simulink model "MTotalRequested"  (R2024b)
settings: Solver=FixedStepAuto  StartTime=0.0  StopTime=10.0  RelTol=1e-3  EnableMultiTasking=on
undefined symbols (not defined in the file): MNominal, MTotalMaxAllowed, MTotalMinAllowed, rGearboxRatio, rTyreRadius
libraries: simulink x4
settings Model: DataDictionary=Master_Dictionary.sldd  EnableAccessToBaseWorkspace=off  Creator=torni  LastModifiedBy=Will
settings OptimizationCC: DefaultParameterBehavior=Inlined  EnhancedBackFolding=on  PassReuseOutputArgsAs=Individual arguments  ZeroExternalMemoryAtStartup=off  ZeroInternalMemoryAtStartup=off  MaxStackSize=8192  OptimizeBlockOrder=speed  DifferentSizesBufferReuse=on  OptimizationCustomize=off  EfficientTunableParamExpr=on
settings DebuggingCC: ParameterTunabilityLossMsg=error
settings HardwareCC: ProdBitPerPointer=32  ProdBitPerSizeT=32  ProdBitPerPtrDiffT=32  ProdLargestAtomicInteger=Long  ProdLargestAtomicFloat=Double  ProdWordSize=32  ProdLongLongMode=on  ProdHWDeviceType=ARM Compatible->ARM Cortex-M
settings SFSimCC: MATLABDynamicMemAlloc=off
settings RTWCC: Description=Embedded Coder  SystemTargetFile=ert.tlc  HardwareBoard=STM32H7xx Based (Single-core)  TemplateMakefile=ert_default_tmf  Toolchain=GNU Tools for ARM Embedded Processors
settings CodeAppCC: ForceParamTrailComments=on  IgnoreCustomStorageClasses=off  OperatorAnnotations=on  SimulinkDataObjDesc=on  SFDataObjDesc=on  InsertBlockDesc=on
settings ERTTargetCC: TargetLangStandard=C99 (ISO)  CodeReplacementLibrary=ARM Cortex-M  ExtModeTransport=3  ExtModeStaticAlloc=on  ExtModeStaticAllocSize=2048  ExtModeMexFile=ext_xcp  ExtModeIntrfLevel=Level2 - Open

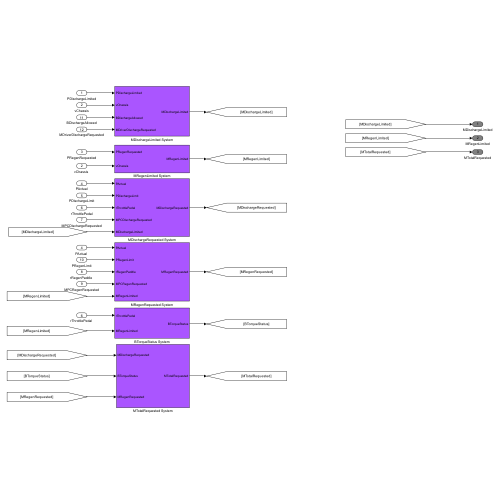
[thumbnail: Simulink's stored preview of the top-level diagram]
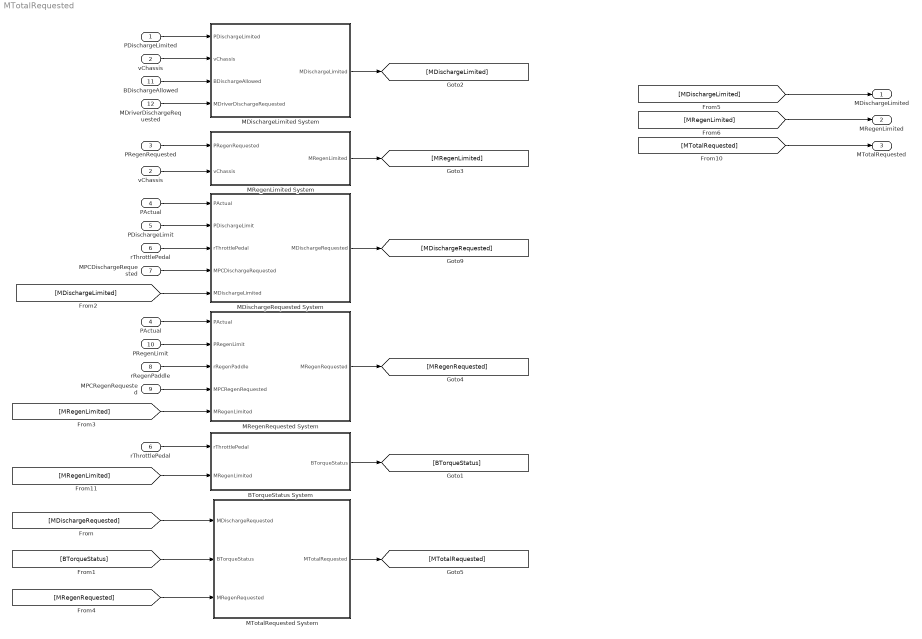
== system MTotalRequested ==
  PDischargeLimited : Inport
  vChassis : Inport  Port=2  OutDataTypeStr=double
  PRegenRequested : Inport  Port=3
  PActual : Inport  Port=4  OutDataTypeStr=double
  PDischargeLimit : Inport  Port=5  OutDataTypeStr=double
  rThrottlePedal : Inport  Port=6  OutDataTypeStr=double
  MPCDischargeRequested : Inport  Port=7  OutDataTypeStr=double
  "rRegenPaddle " : Inport  Port=8  OutDataTypeStr=double
  MPCRegenRequested : Inport  Port=9  OutDataTypeStr=double
  PRegenLimit : Inport  Port=10
  BDischargeAllowed : Inport  Port=11  OutDataTypeStr=boolean
  MDriverDischargeRequested : Inport  Port=12  OutDataTypeStr=double
  BTorqueStatus System : Subsystem
  MDischargeLimited System : Subsystem
  MDischargeRequested System : Subsystem
  MRegenLimited System : Subsystem
  MRegenRequested System : Subsystem
  MTotalRequested System : Subsystem
  "PActual " : InportShadow  Port=4  OutDataTypeStr=double
  "rThrottlePedal " : InportShadow  Port=6  OutDataTypeStr=double
  "vChassis " : InportShadow  Port=2  OutDataTypeStr=double
  MDischargeLimited : Outport  OutDataTypeStr=double  VectorParamsAs1DForOutWhenUnconnected=off
  MRegenLimited : Outport  Port=2  OutDataTypeStr=double  VectorParamsAs1DForOutWhenUnconnected=off
  MTotalRequested : Outport  Port=3  OutDataTypeStr=double  VectorParamsAs1DForOutWhenUnconnected=off
  wires:
  MTotalRequested System/1(MTotalRequested) -> [MTotalRequested]
  BTorqueStatus System/1(BTorqueStatus) -> [BTorqueStatus]
  [BTorqueStatus] -> MTotalRequested System/2(BTorqueStatus)
  rThrottlePedal/1 -> MDischargeRequested System/3(rThrottlePedal)
  [MRegenLimited] -> MRegenRequested System/5(MRegenLimited)
  [MDischargeRequested] -> MTotalRequested System/1(MDischargeRequested)
  PDischargeLimit/1 -> MDischargeRequested System/2(PDischargeLimit)
  [MRegenRequested] -> MTotalRequested System/3(MRegenRequested)
  MRegenRequested System/1(MRegenRequested) -> [MRegenRequested]
  MDischargeLimited System/1(MDischargeLimited) -> [MDischargeLimited]
  MPCRegenRequested/1 -> MRegenRequested System/4(MPCRegenRequested)
  [MRegenLimited] -> BTorqueStatus System/2(MRegenLimited)
  "rRegenPaddle "/1 -> MRegenRequested System/3(rRegenPaddle)
  MRegenLimited System/1(MRegenLimited) -> [MRegenLimited]
  [MDischargeLimited] -> MDischargeRequested System/5(MDischargeLimited)
  PActual/1 -> MDischargeRequested System/1(PActual)
  MDischargeRequested System/1(MDischargeRequested) -> [MDischargeRequested]
  PRegenLimit/1 -> MRegenRequested System/2(PRegenLimit)
  "PActual "/1 -> MRegenRequested System/1(PActual)
  MPCDischargeRequested/1 -> MDischargeRequested System/4(MPCDischargeRequested)
  "rThrottlePedal "/1 -> BTorqueStatus System/1(rThrottlePedal)
  [MTotalRequested] -> MTotalRequested/1
  [MRegenLimited] -> MRegenLimited/1
  [MDischargeLimited] -> MDischargeLimited/1
  PDischargeLimited/1 -> MDischargeLimited System/1(PDischargeLimited)
  vChassis/1 -> MDischargeLimited System/2(vChassis)
  PRegenRequested/1 -> MRegenLimited System/1(PRegenRequested)
  "vChassis "/1 -> MRegenLimited System/2(vChassis)
  BDischargeAllowed/1 -> MDischargeLimited System/3(BDischargeAllowed)
  MDriverDischargeRequested/1 -> MDischargeLimited System/4(MDriverDischargeRequested)

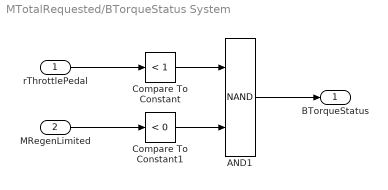
== system MTotalRequested/BTorqueStatus System ==
  rThrottlePedal : Inport  OutDataTypeStr=double
  MRegenLimited : Inport  Port=2  OutDataTypeStr=double
  AND1 : Logic  Operator=NAND  AllPortsSameDT=off  OutDataTypeStr=boolean
  Compare To Constant : simulink/Logic and Bit Operations/Compare To Constant  relop=<  const=1  OutDataTypeStr=boolean
  Compare To Constant1 : simulink/Logic and Bit Operations/Compare To Constant  relop=<  const=0  OutDataTypeStr=boolean
  BTorqueStatus : Outport  OutDataTypeStr=boolean  VectorParamsAs1DForOutWhenUnconnected=off
  wires:
  AND1/1 -> BTorqueStatus/1
  Compare To Constant/1 -> AND1/1
  Compare To Constant1/1 -> AND1/2
  rThrottlePedal/1 -> Compare To Constant/1
  MRegenLimited/1 -> Compare To Constant1/1

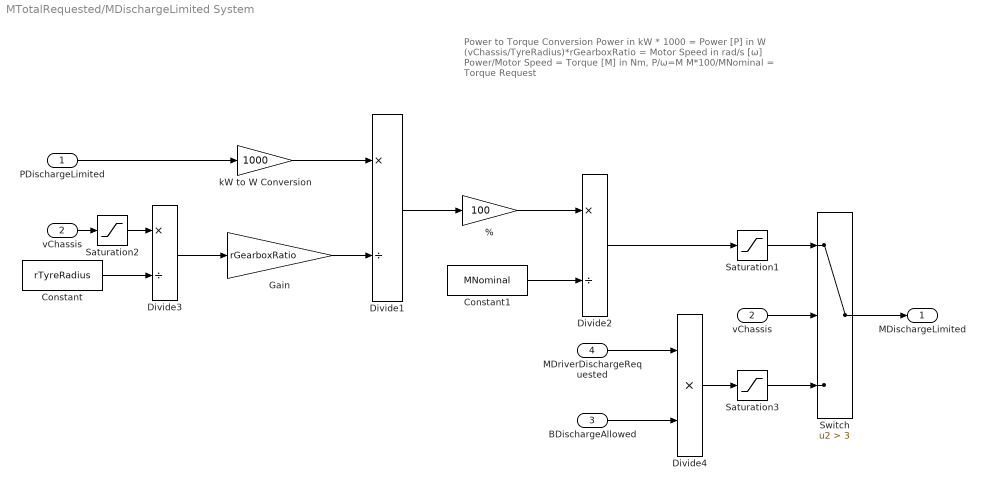
== system MTotalRequested/MDischargeLimited System ==
  note: Power to Torque Conversion
      |
      | Power in kW * 1000 = Power [P] in W
      |
      | (vChassis/TyreRadius)*rGearboxRatio = Motor Speed in rad/s [ω]
      |
      | Power/Motor Speed = Torque [M] in Nm, P/ω=M
      |
      | M*100/MNominal = Torque Request
  PDischargeLimited : Inport
  vChassis : Inport  Port=2  OutDataTypeStr=double
  BDischargeAllowed : Inport  Port=3  OutDataTypeStr=boolean
  MDriverDischargeRequested : Inport  Port=4  OutDataTypeStr=double
  "% " : Gain  Gain=100
  Constant : Constant  Value=rTyreRadius
  Constant1 : Constant  Value=MNominal
  Divide1 : Product  Inputs=*/
  Divide2 : Product  Inputs=*/
  Divide3 : Product  Inputs=*/
  Divide4 : Product  Inputs=**
  Gain : Gain  Gain=rGearboxRatio
  Saturation1 : Saturate  UpperLimit=MTotalMaxAllowed  LowerLimit=0
  Saturation2 : Saturate  UpperLimit=40  LowerLimit=0.1
  Saturation3 : Saturate  UpperLimit=MTotalMaxAllowed  LowerLimit=0
  Switch : Switch  Criteria=u2 > Threshold  Threshold=3  SaturateOnIntegerOverflow=off  InputSameDT=off
  kW to W Conversion : Gain  Gain=1000
  "vChassis " : InportShadow  Port=2  OutDataTypeStr=double
  MDischargeLimited : Outport  OutDataTypeStr=double  VectorParamsAs1DForOutWhenUnconnected=off
  wires:
  PDischargeLimited/1 -> kW to W Conversion/1
  Divide2/1 -> Saturation1/1
  Divide1/1 -> "% "/1
  vChassis/1 -> Saturation2/1
  Constant1/1 -> Divide2/2
  kW to W Conversion/1 -> Divide1/1
  Constant/1 -> Divide3/2
  Switch/1 -> MDischargeLimited/1
  Divide3/1 -> Gain/1
  Gain/1 -> Divide1/2
  "% "/1 -> Divide2/1
  Saturation2/1 -> Divide3/1
  MDriverDischargeRequested/1 -> Divide4/1
  BDischargeAllowed/1 -> Divide4/2
  Saturation1/1 -> Switch/1
  Divide4/1 -> Saturation3/1
  Saturation3/1 -> Switch/3
  "vChassis "/1 -> Switch/2

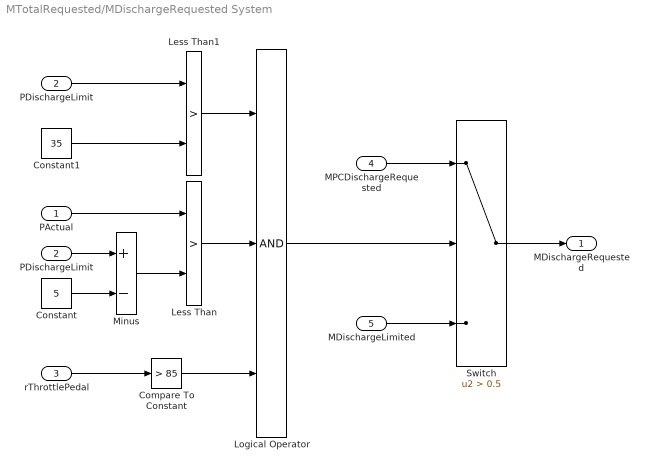
== system MTotalRequested/MDischargeRequested System ==
  PActual : Inport  OutDataTypeStr=double
  PDischargeLimit : Inport  Port=2  OutDataTypeStr=double
  rThrottlePedal : Inport  Port=3  OutDataTypeStr=double
  MPCDischargeRequested : Inport  Port=4  OutDataTypeStr=double
  MDischargeLimited : Inport  Port=5  OutDataTypeStr=double
  Compare To Constant : simulink/Logic and Bit Operations/Compare To Constant  relop=>  const=85  OutDataTypeStr=boolean
  Constant : Constant  Value=5
  Constant1 : Constant  Value=35
  Less Than : RelationalOperator  Operator=>  OutDataTypeStr=boolean  RndMeth=Simplest  InputSameDT=off
  Less Than1 : RelationalOperator  Operator=>  OutDataTypeStr=boolean  RndMeth=Simplest  InputSameDT=off
  Logical Operator : Logic  Inputs=3  AllPortsSameDT=off  OutDataTypeStr=boolean
  Minus : Sum  Inputs=+-
  "PDischargeLimit " : InportShadow  Port=2  OutDataTypeStr=double
  Switch : Switch  Criteria=u2 > Threshold  Threshold=0.5  SaturateOnIntegerOverflow=off  InputSameDT=off
  MDischargeRequested : Outport  OutDataTypeStr=double  VectorParamsAs1DForOutWhenUnconnected=off
  wires:
  Switch/1 -> MDischargeRequested/1
  MDischargeLimited/1 -> Switch/3
  Compare To Constant/1 -> Logical Operator/3
  rThrottlePedal/1 -> Compare To Constant/1
  MPCDischargeRequested/1 -> Switch/1
  Logical Operator/1 -> Switch/2
  PDischargeLimit/1 -> Minus/1
  Constant/1 -> Minus/2
  PActual/1 -> Less Than/1
  Minus/1 -> Less Than/2
  Less Than/1 -> Logical Operator/2
  Less Than1/1 -> Logical Operator/1
  "PDischargeLimit "/1 -> Less Than1/1
  Constant1/1 -> Less Than1/2

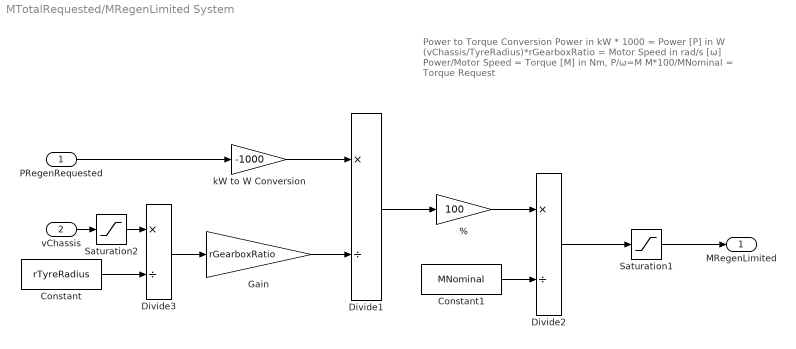
== system MTotalRequested/MRegenLimited System ==
  note: Power to Torque Conversion
      |
      | Power in kW * 1000 = Power [P] in W
      |
      | (vChassis/TyreRadius)*rGearboxRatio = Motor Speed in rad/s [ω]
      |
      | Power/Motor Speed = Torque [M] in Nm, P/ω=M
      |
      | M*100/MNominal = Torque Request
  PRegenRequested : Inport
  vChassis : Inport  Port=2  OutDataTypeStr=double
  "% " : Gain  Gain=100
  Constant : Constant  Value=rTyreRadius
  Constant1 : Constant  Value=MNominal
  Divide1 : Product  Inputs=*/
  Divide2 : Product  Inputs=*/
  Divide3 : Product  Inputs=*/
  Gain : Gain  Gain=rGearboxRatio
  Saturation1 : Saturate  UpperLimit=0  LowerLimit=MTotalMinAllowed
  Saturation2 : Saturate  UpperLimit=40  LowerLimit=0.1
  kW to W Conversion : Gain  Gain=-1000
  MRegenLimited : Outport  OutDataTypeStr=double  VectorParamsAs1DForOutWhenUnconnected=off
  wires:
  PRegenRequested/1 -> kW to W Conversion/1
  Divide2/1 -> Saturation1/1
  Divide1/1 -> "% "/1
  vChassis/1 -> Saturation2/1
  Constant1/1 -> Divide2/2
  kW to W Conversion/1 -> Divide1/1
  Constant/1 -> Divide3/2
  Saturation1/1 -> MRegenLimited/1
  "% "/1 -> Divide2/1
  Divide3/1 -> Gain/1
  Gain/1 -> Divide1/2
  Saturation2/1 -> Divide3/1

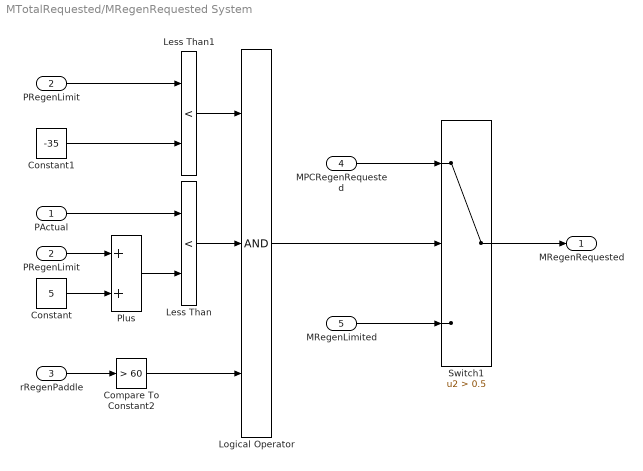
== system MTotalRequested/MRegenRequested System ==
  PActual : Inport  OutDataTypeStr=double
  PRegenLimit : Inport  Port=2  OutDataTypeStr=double
  rRegenPaddle : Inport  Port=3  OutDataTypeStr=double
  MPCRegenRequested : Inport  Port=4  OutDataTypeStr=double
  MRegenLimited : Inport  Port=5  OutDataTypeStr=double
  Compare To Constant2 : simulink/Logic and Bit Operations/Compare To Constant  relop=>  const=60  OutDataTypeStr=boolean
  Constant : Constant  Value=5
  Constant1 : Constant  Value=-35
  Less Than : RelationalOperator  Operator=<  OutDataTypeStr=boolean  RndMeth=Simplest  InputSameDT=off
  Less Than1 : RelationalOperator  Operator=<  OutDataTypeStr=boolean  RndMeth=Simplest  InputSameDT=off
  Logical Operator : Logic  Inputs=3  AllPortsSameDT=off  OutDataTypeStr=boolean
  "PRegenLimit " : InportShadow  Port=2  OutDataTypeStr=double
  Plus : Sum
  Switch1 : Switch  Criteria=u2 > Threshold  Threshold=0.5  SaturateOnIntegerOverflow=off  InputSameDT=off
  MRegenRequested : Outport  OutDataTypeStr=double  VectorParamsAs1DForOutWhenUnconnected=off
  wires:
  Switch1/1 -> MRegenRequested/1
  MPCRegenRequested/1 -> Switch1/1
  MRegenLimited/1 -> Switch1/3
  rRegenPaddle/1 -> Compare To Constant2/1
  Logical Operator/1 -> Switch1/2
  Compare To Constant2/1 -> Logical Operator/3
  PActual/1 -> Less Than/1
  Plus/1 -> Less Than/2
  PRegenLimit/1 -> Plus/1
  Constant/1 -> Plus/2
  Less Than/1 -> Logical Operator/2
  Less Than1/1 -> Logical Operator/1
  "PRegenLimit "/1 -> Less Than1/1
  Constant1/1 -> Less Than1/2

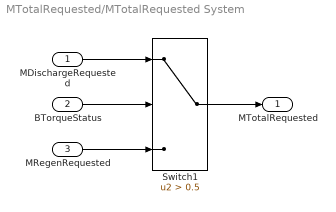
== system MTotalRequested/MTotalRequested System ==
  MDischargeRequested : Inport  OutDataTypeStr=double
  BTorqueStatus : Inport  Port=2  OutDataTypeStr=boolean
  MRegenRequested : Inport  Port=3  OutDataTypeStr=double
  Switch1 : Switch  Criteria=u2 > Threshold  Threshold=0.5  SaturateOnIntegerOverflow=off  InputSameDT=off
  MTotalRequested : Outport  OutDataTypeStr=double  VectorParamsAs1DForOutWhenUnconnected=off
  wires:
  Switch1/1 -> MTotalRequested/1
  MDischargeRequested/1 -> Switch1/1
  BTorqueStatus/1 -> Switch1/2
  MRegenRequested/1 -> Switch1/3
